simulink model "simulator"  (R2024b)
settings: Solver=ode4  StartTime=0.0  StopTime=inf  RelTol=1e-3
values from neighbouring files (symbols this model uses):
  FlowBoost = 100    [init.m]
  h = 4    [init.m]
  InitialLevel = 2.0    (= 2)    [init.m]
  qOut_median = 16.6/3600    (= 0.00461111111111)    [init.m]
  qOut_simAmplitude = (qOut_usualMax - qOut_usualMin)/2    (= 0.00184722222222)    [init.m]
  qV_max = 50/3600    (= 0.0138888888889)    [init.m]
undefined symbols (not defined in the file or in its folder): daq
libraries: daqlib x2, instrumentlib x1
settings Model: Creator=antho  LastModifiedBy=antho

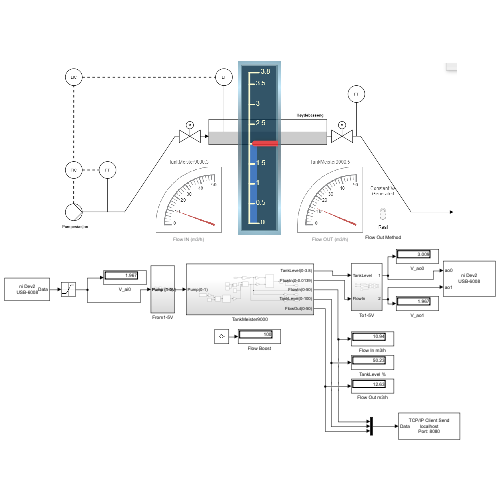
[thumbnail: Simulink's stored preview of the top-level diagram]
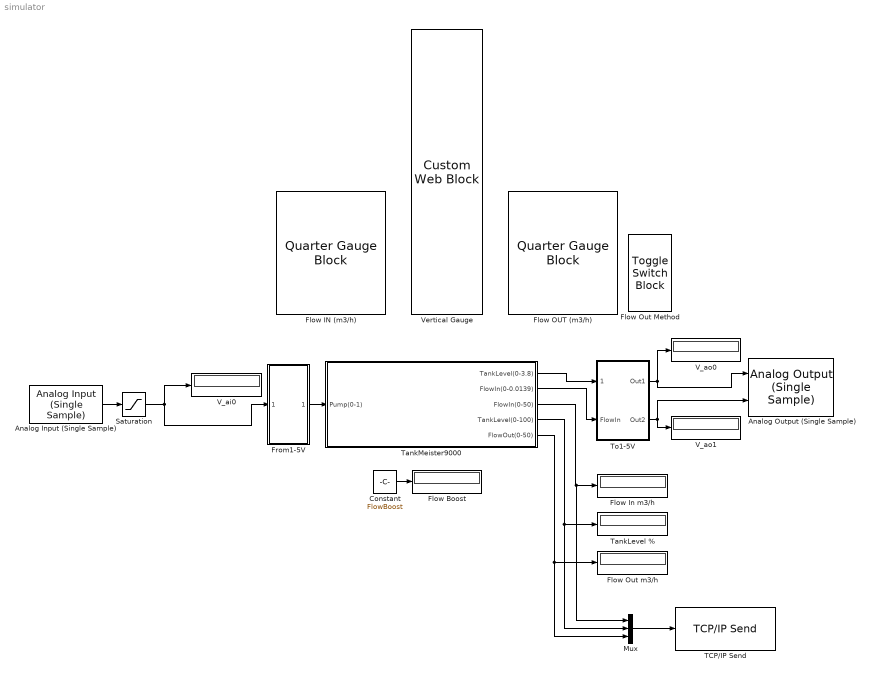
== system simulator ==
  Analog Input (Single Sample) : daqlib/Analog Input (Single Sample)  DeviceMenu=ni Dev2 (USB-6008)  Device=ni Dev2 (USB-6008)  ObjConstructor=daq.createSession('ni')  BlockSampleTime=1  NChannelsSelected=1  Channels=1$ai0$$Dev2$1$6$1$1$#0$ai1$$Dev2$1$1$1$1$#0$ai2$$Dev2$1$1$1$1$#0$ai3$$Dev2$1$1$1$1$#0$ai4$$Dev2$1$1$1$1$#0$ai5$$Dev2$1$1$1$1$#0$ai6$$Dev2$1$1$1$1$#0$ai7$$Dev2$1$1$1$1$#  NPorts=1 for all channels  OutputTimestamp=off
  Analog Output (Single Sample) : daqlib/Analog Output (Single Sample)  DeviceMenu=ni Dev2 (USB-6008)  Device=ni Dev2 (USB-6008)  ObjConstructor=daq.createSession('ni')  NChannelsSelected=2  Channels=1$ao0$$Dev2$1$1$N/A$#1$ao1$$Dev2$1$1$N/A$#  NPorts=1 per channel  BlockSampleTime=1
  Constant : Constant  Value=FlowBoost
  Flow Boost : Display
  Flow IN (m3/h) : QuarterGaugeBlock  ScaleMax=50
  Flow In m3/h : Display
  Flow OUT (m3/h) : QuarterGaugeBlock  ScaleMax=50
  Flow Out Method : ToggleSwitchBlock
      settings: Values={{'Real', 'Generated'}, [0 1]}
  Flow Out m3/h : Display
  From1-5V : Subsystem
  Mux : Mux  Inputs=3
  Saturation : Saturate  UpperLimit=5  LowerLimit=1
  TCP/IP Send : instrumentlib/TCP//IP Send  Host=localhost  Port=8080  ByteOrder=little-endian  EnableBlockingMode=off  Timeout=10  TransferDelay=off  SimulateUsing=Interpreted execution
  TankLevel % : Display
  TankMeister9000 : Subsystem
  To1-5V : Subsystem
  V_ai0 : Display
  V_ao0 : Display
  V_ao1 : Display
  Vertical Gauge : CustomWebBlock  LabelPosition=Hide  ShowInitialText=on  Configuration="{\"components\":[{\"name\":\"LinearScaleComponent\",\"settings\":{\"bounds\":{\"max\":3.8,\"min\":0,\"tickInterval\":\"auto\"},\"internalTickHeightScaleFactor\":0.5,\"labelColor\":[255,255,200],\"labelFont\":{\"font\":\"Arial\",\"fontSize\":12},\"labelOffset\":0.05,\"labelTransparency\":1,\"needleImage\":{\"size\":[21,75],\"src\":\"data:image\\/svg+xml;base64,PHN2ZyB4bWxucz0iaHR0cDovL3d3dy53My5vcmcvMjAwMC9zdmciIHhtbG5zOnhsaW5rPSJodHRwOi8vd3d3LnczLm9yZy8xOTk5L3hsaW5rIiB2aWV3Qm94PSIwIDAgMjEgNzUiPjxkZWZzPjxzdHlsZT4uY2xzLTF7ZmlsbDpub25lO30uY2xzLTJ7aXNvbGF0aW9uOmlzb2xhdGU7fS5jbHMtM3tjbGlwLXBhdGg6dXJsKCNjbGlwLXBhdGgpO30uY2xzLTR7b3BhY2l0eTowLjM7bWl4LWJsZW5kLW1vZGU6bXVsdGlwbHk7fS5jbHMtNXtmaWxsOiNlYjI2Mjk7fTwvc3R5bGU+PGNsaXBQYXRoIGlkPSJjbGlwLXBhdGgiIHRyYW5zZm9y ...(+1928 chars)\",\"srcOrientation\":\"horizontal\"},\"needleOffset\":[0.007413509060955519,0],\"needleSize\":{\"height\":0.11955094537815127,\"width\":0.7589285714285714},\"position\":[0.015821953781512604,0.06944444444444445,0.7996031746031746,0.9641544117647058],\"referencePoint\":\"auto\",\"scaleColors\":[],\"scaleColorsSize\":0.2,\"scaleDirection\":\"BT\",\"showLabels\":1,\"showMinorTicks\":0,\"showSpanLine\":1,\"showTicks\":1,\"tickColor\":[252,252,197],\"tickTransparency\":1,\"valueBarColor\":[23,89,176],\"valueBarOffset\":0,\"valueBarSize\":0.23,\"valueBarTransparency\":1}},{\"name\":\"BackgroundImageComponent\",\"settings\":{\"image\":{\"size\":[380,101],\"src\":\"data:image\\/svg+xml;base64,PHN2ZyBpZD0iZnJhbWUiIHhtbG5zPSJodHRwOi8vd3d3LnczLm9yZy8yMDAwL3N2ZyIgeG1sbnM6eGxpbms9Imh0dHA6Ly93d3cudzMub3JnLzE5OTkveGxpbmsiIHZpZXdCb3g9IjAgMCAzODAgMTAxIj48ZGVmcz48c3R5bGU+LmNscy0xe2ZpbGw6IzAwMmI0Mjt9LmNscy0ye2ZpbGw6IzQyNzA4Mjt9LmNscy0ze2ZpbGw6dXJsKCNyYWRpYWwtZ3JhZGllbnQpO308L3N0eWxlPjxyYWRpYWxHcmFkaWVudCBpZD0icmFkaWFsLWdyYWRpZW50IiBjeD0iMTkwIiBjeT0iNTAuNSIgcj0iMjY5LjIxIiBncmFkaWVudFVuaXRzPSJ1c2VyU3BhY2VPblVzZSI+PHN0b3Agb2Zmc2V0PSIwLjAxIiBzdG9wLWNvbG9yPSIjM2U0ZjU4Ii8+PHN0b3Agb2Zmc2V0PSIwLjA2IiBzdG9wLWNvbG9yPSIjNDQ1NzYxIi8+PHN0b3Agb2Zmc2V0PSIwLjE1IiBzdG9wLWNvbG9yPSIjNTU2YTc2Ii8+PHN0b3Agb2Zmc2V0PSIwLjI1IiBzdG9wLWNvbG9yPSIjNmQ4ODk1Ii8+PHN0b3Agb2Zmc2V0PSIwLjM4IiBzdG9wLWNvbG9yPSIjOGZiMmMzIi8+PHN0b3Agb2Zmc2V0PSIwLjUyIiBzdG9wLWNvbG9yPSIjYjZlNGZhIi8+PHN0b3Agb2Zmc2V0PSIxIiBzdG9wLWNvbG9yPSIjMTU0NjU3Ii8+PC9yYWRpYWxHcmFkaWVudD48L2RlZnM+PGcgaWQ9IkxheWVyXzIiIGRhdGEtbmFtZT0iTGF5ZXIgMiI+PGcgaWQ9IkxheWVyXzEtMiIgZGF0YS1uYW1lPSJMYXllciAxLTIiPjxyZWN0IGlkPSJyZWN0MTAzNiIgY2xhc3M9ImNscy0xIiB4PSIxMSIgeT0iMTEiIHdpZHRoPSIzNTgiIGhlaWdodD0iNzkiLz48cGF0aCBpZD0icGF0aDEwMzgiIGNsYXNzPSJjbHMtMiIgZD0iTTgsOFY5M0gzNzJWOFpNMzY5LDkwSDExVjExSDM2OVoiLz48cGF0aCBpZD0icGF0aDEwNDAiIGNsYXNzPSJjbHMtMyIgZD0iTTAsMFYxMDFIMzgwVjBaTTM3Miw5M0g4VjhIMzcyWiIvPjwvZz48L2c+PC9zdmc+\",\"srcOrientation\":\"horizontal\"},\"position\":[0,0,1,1],\"scaleMode\":\"0\"}},{\"name\":\"ForegroundImageComponent\",\"settings\":{\"image\":{\"size\":[0,0],\"src\":\"default\",\"srcOrientation\":[]},\"isForeground\":1,\"position\":[0,0,1,1],\"scaleMode\":\"0\"}}],\"settings\":{\"BindingType\":\"signal\",\"backgroundColor\":[0,0,0,\"1\"],\"backgroundOffset\":0,\"backgroundOpacity\":1,\"fixedAspectRatio\":\"on\",\"orientation\":\"vertical\",\"showBackgroundColor\":false,\"value\":0,\"version\":\"R2023a\"},\"type\":\"LinearGauge\"}"
  wires:
  TankMeister9000/1(TankLevel(0-3.8)) -> To1-5V/1(TankLevel)
  TankMeister9000/2(FlowIn(0-0.0139)) -> To1-5V/2(FlowIn)
  From1-5V/1(Pump (1-0)) -> TankMeister9000/1(Pump(0-1))
  To1-5V/1(Out1) -> V_ao0/1, Analog Output (Single Sample)/1
  To1-5V/2(Out2) -> Analog Output (Single Sample)/2, V_ao1/1
  TankMeister9000/4(TankLevel(0-100)) -> Mux/2, TankLevel %/1
  Constant/1 -> Flow Boost/1
  TankMeister9000/3(FlowIn(0-50)) -> Mux/1, Flow In m3/h/1
  TankMeister9000/5(FlowOut(0-50)) -> Mux/3, Flow Out m3/h/1
  Analog Input (Single Sample)/1 -> Saturation/1
  Saturation/1 -> From1-5V/1(Pump (1-5V)), V_ai0/1
  Mux/1 -> TCP/IP Send/1

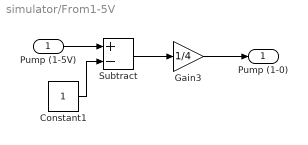
== system simulator/From1-5V ==
  Pump (1-5V) : Inport
  Constant1 : Constant
  Gain3 : Gain  Gain=1/4
  Subtract : Sum  Inputs=+-
  Pump (1-0) : Outport
  wires:
  Constant1/1 -> Subtract/2
  Pump (1-5V)/1 -> Subtract/1
  Subtract/1 -> Gain3/1
  Gain3/1 -> Pump (1-0)/1

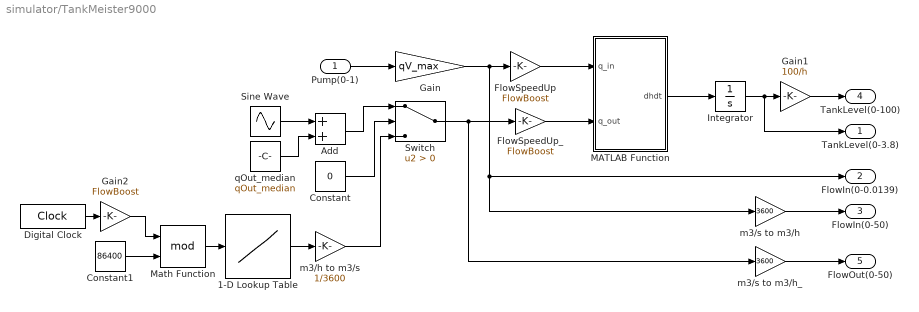
== system simulator/TankMeister9000 ==
  Pump(0-1) : Inport
  1-D Lookup Table : Lookup_n-D  NumberOfTableDimensions=1  BreakpointsForDimension1=[0;288;576;864;1152;1440;1728;2016;2304;2592;2880;3168;3456;3744;4032;4320;4608;4896;5184;5472;5760;6048;6336;6624;6912;7200;7488;7776;8064;8352;8640;8928;9216;9504;9792;10080;10368;10656;10944;11232;11520;11808;12096;12384;12672;12960;13248;13536;13824;14112;14400;14688;14976;15264;15552;15840;16128;16416;16704;16992;17280;17568;17856;18144;18432;18720;19008;19296;19584;19872;20160;20448;20736;21024;21312;21600;21888;22176;22464;22752;23040;23328;23616;23904;24192;24480;24768;25056;25344;25632;25920;26208;26496;26784;27072;27360;27648;27936;28224;28512;28800;29088;29376;29664;29952;30240;30528;30816;31104;31392;31680;31968;32256;32544;32832;33120;33408;33696;33984;34272;34560;34848;35136;35424;35712;36000;36288;36576;36864;37152;37440;37728;38016;38304;38592;38880;39168;39456;39744;40032;40320;40608;40896;41184;41472;41760;42048;42336;42624;42912;43200;43488;43776;44064;44352;44640;44928;45216;45504;45792;46080;46368;46656;46944;47232;47520;47808;48096;48384;48672;48960;49248;49536;49824;50112;50400;50688;50976;51264;51552;51840;52128;52416;52704;52992;53280;53568;53856;54144;54432;54720;55008;55296;55584;55872;56160;56448;56736;57024;57312;57600;57888;58176;58464;58752;59040;59328;59616;59904;60192;60480;60768;61056;61344;61632;61920;62208;62496;62784;63072;63360;63648;63936;64224;64512;64800;65088;65376;65664;65952;66240;66528;66816;67104;67392;67680;67968;68256;68544;68832;69120;69408;69696;69984;70272;70560;70848;71136;71424;71712;72000;72288;72576;72864;73152;73440;73728;74016;74304;74592;74880;75168;75456;75744;76032;76320;76608;76896;77184;77472;77760;78048;78336;78624;78912;79200;79488;79776;80064;80352;80640;80928;81216;81504;81792;82080;82368;82656;82944;83232;83520;83808;84096;84384;84672;84960;85248;85536;85824;86112;86400]  Table=[16.2841516;16.5673652;16.308551;17.4394106;19.1363052;18.7597848;17.7330304;16.9856068;16.6888823;17.3544765;17.8218263;18.1274955;18.2209805;18.64702;18.6778833;18.5444921;18.1540753;17.62776;18.326131;18.2694705;17.902114;17.244003;16.6657269;17.819349;19.1239116;19.4737452;18.6103761;18.3200866;18.6669026;18.7781972;18.1294632;18.3681507;19.5541061;19.4851681;19.5704582;20.2541194;20.5368896;20.9539653;20.7811564;19.6248132;18.2136619;16.7741547;17.023907;19.2258518;20.8231253;20.5268467;19.4978461;18.3659207;18.2108725;18.6435625;18.507381;19.3901992;19.6500007;19.2884231;19.4959406;18.6798435;19.3896156;20.0574955;18.9097385;19.2826362;18.7395015;17.9703698;19.3524822;19.5367941;19.3763154;19.0666091;18.5780936;19.2180524;19.7405619;18.9111336;18.5752398;19.2124683;18.8619435;18.6418699;18.4530323;18.0804711;17.3893407;17.0149937;17.5748537;16.7794942;15.8496637;15.6121936;15.9549328;16.2301057;15.5743217;15.6410735;16.5481941;16.4859893;15.6639723;16.6731375;17.2297374;16.5423702;15.8889033;16.2731585;15.6735578;14.7521296;14.9239527;15.0799918;14.8453531;15.0917483;15.8498832;16.7157442;18.2455621;17.6316403;17.2855054;16.8078614;16.2810157;16.0538004;16.1375022;17.1401293;17.1338307;16.8125463;17.131819;17.5981852;17.6420258;16.5158103;16.1572953;16.7186619;15.8168736;14.7743127;14.6626081;15.4036427;16.3835674;15.2647496;13.9620744;15.0669903;16.1619922;15.9690256;14.6450966;13.9080002;14.5489559;13.6864875;13.0868047;12.8093342;12.6297854;13.5946618;14.1911243;13.5650456;13.1927007;13.4423878;13.3270876;12.8986606;13.12481;12.9644516;12.2359157;12.2402356;11.9819549;12.0711234;12.2750588;11.8478548;11.6998997;11.6309219;11.5984204;11.6771508;11.413089;11.0589607;11.1426696;11.2975537;11.564722;11.5874638;11.2683062;10.8727691;10.622348;10.7176887;11.2762551;11.8359576;11.7593106;11.7710462;11.3762746;11.0391551;11.1385055;11.1320349;11.1630802;11.402946;11.2991164;11.1460673;11.2666657;11.4402381;11.430663;11.4406865;11.261325;11.4471425;11.6993222;11.7772867;11.782155;11.513712;11.6163338;11.8259206;11.6295876;11.7253632;11.7431233;11.8944089;12.080291;12.6047028;13.0131603;12.4682277;12.4979947;12.7433897;12.5109342;12.278746;12.2555549;11.9536222;12.1853159;12.5289597;12.8991419;13.2548247;13.0480204;12.7827043;12.9886571;13.2604638;13.4268656;13.8688365;13.6505638;14.272972;14.441021;13.5406179;13.3445494;14.0160649;14.9311;15.6505883;15.5971581;16.2090287;17.2706335;19.1589002;19.8925164;19.0418291;18.7442756;18.7819998;19.1660375;19.4266846;17.2667559;17.7338952;19.5968549;18.9274362;19.5439502;19.7783399;20.3714066;22.1715311;21.2703969;20.2400204;20.1586112;20.2346961;20.6073272;21.7293089;21.3210315;20.9050579;21.0915484;22.158941;23.6602811;23.8931757;22.4521598;20.1352647;20.6771874;20.9521092;20.7580465;21.6024225;20.1733932;20.1384313;22.0127632;21.1596288;20.7288166;21.2847702;21.1278761;20.2967851;20.3568968;20.3597684;19.3619695;19.251405;19.8947585;20.1198302;19.8665567;19.6809373;20.3142474;20.1112406;19.5623763;20.5753765;20.882822;19.0894664;18.1640065;19.1169365;19.5645786;19.7386063;18.6457691;17.4848411;17.0944964;17.1266768;18.2124536;18.0525692;19.3028121;19.7553775;18.21817;17.3735058;18.427342;18.486639;19.2745191;19.4038482;19.0263262;19.8457628;17.659274;16.5981011;20.6062508]  InternalRulePriority=Speed  RndMeth=Simplest
  Add : Sum
  Constant : Constant  Value=0
  Constant1 : Constant  Value=86400
  Digital Clock : DigitalClock
  FlowSpeedUp : Gain  Gain=FlowBoost
  FlowSpeedUp_ : Gain  Gain=FlowBoost
  Gain : Gain  Gain=qV_max
  Gain1 : Gain  Gain=100/h
  Gain2 : Gain  Gain=FlowBoost
  Integrator : Integrator  InitialCondition=InitialLevel  LimitOutput=on  UpperSaturationLimit=h  LowerSaturationLimit=0
  MATLAB Function : MATLAB Function  TreatAsAtomicUnit=on
  Math Function : Math  Operator=mod
  Sine Wave : Sin  Amplitude=qOut_simAmplitude  Frequency=0.1  SampleTime=0
  Switch : Switch  Criteria=u2 > Threshold  SaturateOnIntegerOverflow=off  InputSameDT=off
  m3/h to m3/s : Gain  Gain=1/3600
  m3/s to m3/h : Gain  Gain=3600
  m3/s to m3/h_ : Gain  Gain=3600
  qOut_median : Constant  Value=qOut_median
  TankLevel(0-3.8) : Outport
  FlowIn(0-0.0139) : Outport  Port=2
  FlowIn(0-50) : Outport  Port=3
  TankLevel(0-100) : Outport  Port=4
  FlowOut(0-50) : Outport  Port=5
  wires:
  qOut_median/1 -> Add/2
  Integrator/1 -> TankLevel(0-3.8)/1, Gain1/1
  MATLAB Function/1(dhdt) -> Integrator/1
  Pump(0-1)/1 -> Gain/1
  Gain/1 -> FlowSpeedUp/1, m3/s to m3/h/1, FlowIn(0-0.0139)/1
  Gain1/1 -> TankLevel(0-100)/1
  FlowSpeedUp/1 -> MATLAB Function/1(q_in)
  FlowSpeedUp_/1 -> MATLAB Function/2(q_out)
  m3/s to m3/h/1 -> FlowIn(0-50)/1
  m3/s to m3/h_/1 -> FlowOut(0-50)/1
  Sine Wave/1 -> Add/1
  Switch/1 -> m3/s to m3/h_/1, FlowSpeedUp_/1
  Add/1 -> Switch/1
  Constant/1 -> Switch/2
  Constant1/1 -> Math Function/2
  Math Function/1 -> 1-D Lookup Table/1
  Digital Clock/1 -> Gain2/1
  Gain2/1 -> Math Function/1
  1-D Lookup Table/1 -> m3/h to m3/s/1
  m3/h to m3/s/1 -> Switch/3

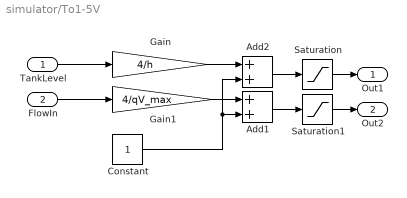
== system simulator/To1-5V ==
  TankLevel : Inport
  FlowIn : Inport  Port=2
  Add1 : Sum
  Add2 : Sum
  Constant : Constant
  Gain : Gain  Gain=4/h
  Gain1 : Gain  Gain=4/qV_max
  Saturation : Saturate  UpperLimit=5  LowerLimit=1
  Saturation1 : Saturate  UpperLimit=5  LowerLimit=1
  Out1 : Outport
  Out2 : Outport  Port=2
  wires:
  FlowIn/1 -> Gain1/1
  Constant/1 -> Add1/2, Add2/2
  Gain1/1 -> Add1/1
  Gain/1 -> Add2/1
  TankLevel/1 -> Gain/1
  Add1/1 -> Saturation1/1
  Saturation1/1 -> Out2/1
  Saturation/1 -> Out1/1
  Add2/1 -> Saturation/1

== matlab function simulator/TankMeister9000/MATLAB Function ==
  data: dhdt output; q_in input; q_out input; A parameter
function dhdt = TankLevel(q_in,q_out, A)

dhdt = (1/A)*(q_in-q_out);
